simulink model "CFBTTCQIED"  (R2021b)
settings: Solver=ode23t  StartTime=0.0  StopTime=simtime  RelTol=1e-3
values from neighbouring files (symbols this model uses):
  a1 = (Iyy-Izz)/Ixx    (= -0.733333333333)    [CFBTTCQIED.m]
  a1_p = 1    [CFBTTCQIED.m]
  a1_r = 1    [CFBTTCQIED.m]
  a1_x = 1    [CFBTTCQIED.m]
  a1_y = 1    [CFBTTCQIED.m]
  a1_z = 1    [CFBTTCQIED.m]
  a2 = Jr/Ixx    (= 0.008)    [CFBTTCQIED.m]
  a2_r = 2    [CFBTTCQIED.m]
  a2_x = 2    [CFBTTCQIED.m]
  a2_y = 2    [CFBTTCQIED.m]
  a2_z = 2    [CFBTTCQIED.m]
  a3 = (Izz-Ixx)/Iyy    (= 0.733333333333)    [CFBTTCQIED.m]
  a4 = Jr/Iyy    (= 0.008)    [CFBTTCQIED.m]
  a5 = (Ixx-Iyy)/Izz    (= 0)    [CFBTTCQIED.m]
  b = 3.13e-5    (= 3.13e-05)    [CFBTTCQIED.m]
  b1 = l/Ixx    (= 30.6666666667)    [CFBTTCQIED.m]
  b2 = l/Iyy    (= 30.6666666667)    [CFBTTCQIED.m]
  b3 = l/Izz    (= 17.6923076923)    [CFBTTCQIED.m]
  d = 7.5e-7    (= 7.5e-07)    [CFBTTCQIED.m]
  epsi = 0.00001    (= 1e-05)    [CFBTTCQIED.m]
  g = 9.81    [CFBTTCQIED.m]
  init_cond_pitch = 0    [CFBTTCQIED.m]
  init_cond_roll = 0    [CFBTTCQIED.m]
  init_cond_x = 0    [CFBTTCQIED.m]
  init_cond_y = 2    [CFBTTCQIED.m]
  init_cond_yaw = 0    [CFBTTCQIED.m]
  init_cond_z = 0    [CFBTTCQIED.m]
  k = 2.980e-6    (= 2.98e-06)    [CFBTTCQIED.m]
  lambda = zxc    (= 10)    [CFBTTCQIED.m]
  lambda_x = 2    [CFBTTCQIED.m]
  lambda_y = 2    [CFBTTCQIED.m]
  lambda_z = 2    [CFBTTCQIED.m]
  lamda_phi = zxc    (= 10)    [CFBTTCQIED.m]
  lamda_psi = zxc    (= 10)    [CFBTTCQIED.m]
  lamda_theta = zxc    (= 10)    [CFBTTCQIED.m]
  m = 0.650    (= 0.65)    [CFBTTCQIED.m]
  Omega_r = 1    [CFBTTCQIED.m]
  p1_phi = 20    [CFBTTCQIED.m]
  p1_psi = 20    [CFBTTCQIED.m]
  p1_theta = 20    [CFBTTCQIED.m]
  p1_x = 2    [CFBTTCQIED.m]
  p1_y = 2    [CFBTTCQIED.m]
  p1_z = 2    [CFBTTCQIED.m]
  p2_phi = 5    [CFBTTCQIED.m]
  p2_psi = 5    [CFBTTCQIED.m]
  p2_theta = 5    [CFBTTCQIED.m]
  p2_x = 2    [CFBTTCQIED.m]
  p2_y = 2    [CFBTTCQIED.m]
  p2_z = 2    [CFBTTCQIED.m]
  psi_des = yaw_des    (= 0.523598775598)    [CFBTTCQIED.m]
  sample_time_pitch = 15    [CFBTTCQIED.m]
  sample_time_roll = 15    [CFBTTCQIED.m]
  sample_time_yaw = 1    [CFBTTCQIED.m]
  tau = 0.1    [CFBTTCQIED.m]
libraries: simulink x2
(part 1 of 2)
settings Model: Creator=nigarahmed  LastModifiedBy=Nigar

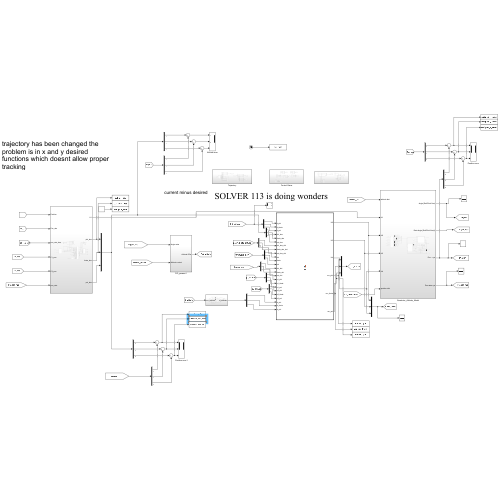
[thumbnail: Simulink's stored preview of the top-level diagram]
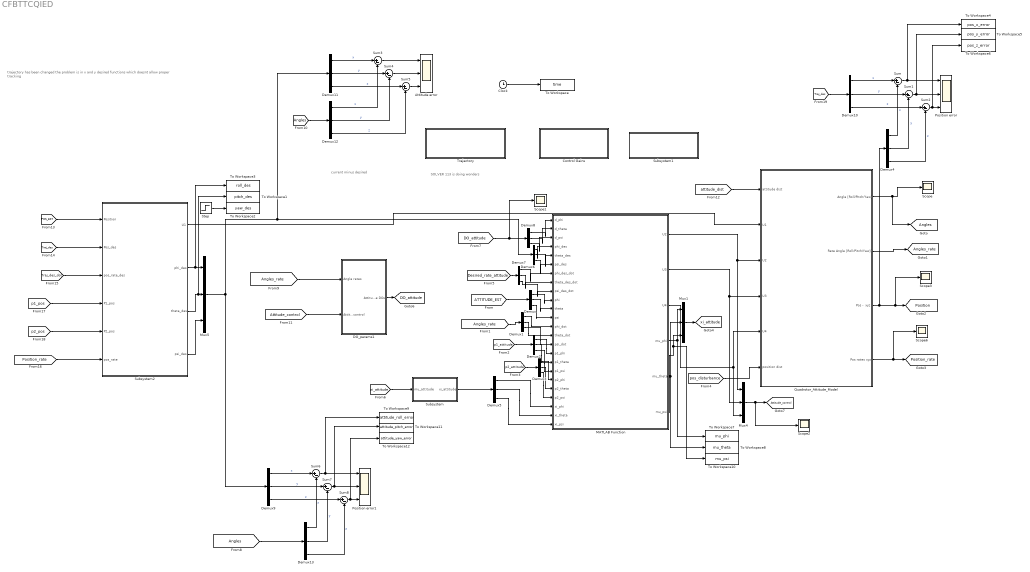
== system CFBTTCQIED ==
  note: current minus desired
  note: SOLVER 113 is doing wonders
  note: trajectory has been changed the problem is in x and y desired functions which doesnt allow proper tracking
  Attitude error : Scope  NumInputPorts=3
  Clock : Clock
  Control Gains : Subsystem
  DO_params1 : Subsystem
  Demux{,1..13} (14 alike) : Demux  Outputs=3
  MATLAB Function : MATLAB Function  TreatAsAtomicUnit=on
  Mux1 : Mux  Inputs=3
  Mux4 : Mux  Inputs=3
  Mux5 : Mux  Inputs=3
  Position error : Scope  NumInputPorts=3
  Position error1 : Scope  NumInputPorts=3
  Quadrotor_Attitude_Model : Subsystem
  Scope{,1..3,6} (5 alike) : Scope
  Step : Step  Time=0  After=psi_des  SampleTime=0
  Subsystem : Subsystem
  Subsystem1 : Subsystem
  Subsystem2 : Subsystem
  Sum{,1..8} (9 alike) : Sum  Inputs=|+-
  To Workspace : ToWorkspace  VariableName=time  SampleTime=-1
  To Workspace1 : ToWorkspace  VariableName=pitch_des  SampleTime=-1
  To Workspace10 : ToWorkspace  VariableName=mu_psi  SampleTime=-1
  To Workspace11 : ToWorkspace  VariableName=attitude_pitch_error  SampleTime=-1
  To Workspace12 : ToWorkspace  VariableName=attitude_yaw_error  SampleTime=-1
  To Workspace2 : ToWorkspace  VariableName=yaw_des  SampleTime=-1
  To Workspace3 : ToWorkspace  VariableName=roll_des  SampleTime=-1
  To Workspace4 : ToWorkspace  VariableName=pos_x_error  SampleTime=-1
  To Workspace5 : ToWorkspace  VariableName=pos_y_error  SampleTime=-1
  To Workspace6 : ToWorkspace  VariableName=pos_z_error  SampleTime=-1
  To Workspace7 : ToWorkspace  VariableName=mu_phi  SampleTime=-1
  To Workspace8 : ToWorkspace  VariableName=mu_theta  SampleTime=-1
  To Workspace9 : ToWorkspace  VariableName=attitude_roll_error  SampleTime=-1
  Trajectory : Subsystem
  tag scope: Angles=global, Angles_rate=global, Attitude_control=global, DO_attitude=global, Position=global, Position_rate=global, xi_attitude=global
  wires:
  [p1_pos] -> Subsystem2/4(P1_pos)
  Quadrotor_Attitude_Model/4(Pos rates xyz) -> Scope6/1, [Position_rate]
  Sum2/1 -> To Workspace6/1, Position error/3
  [Angles_rate] -> DO_params1/1(Angle rates)
  Quadrotor_Attitude_Model/1(Angle [Roll/Pitch/Yaw]) -> [Angles], Scope/1
  DO_params1/1(Attitude DOs) -> [DO_attitude]
  Demux4/3 -> Sum2/2  "z"
  Sum/1 -> To Workspace4/1, Position error/1
  Demux10/2 -> Sum1/1  "y"
  Demux6/2 -> MATLAB Function/5(theta_des)
  [DO_attitude] -> Demux8/1, Scope1/1
  Demux/2 -> MATLAB Function/11(theta)
  Demux4/1 -> Sum/2  "x"
  Demux3/1 -> MATLAB Function/19(p2_phi)
  Demux10/3 -> Sum2/1  "z"
  Demux5/3 -> MATLAB Function/24(xi_psi)
  Demux8/3 -> MATLAB Function/3(d_psi)
  [POS_EST] -> Subsystem2/1(Position)
  Demux6/1 -> MATLAB Function/4(phi_des)
  [Angles_rate] -> Demux1/1
  Demux/1 -> MATLAB Function/10(phi)
  Demux1/3 -> MATLAB Function/15(psi_dot)
  Demux3/2 -> MATLAB Function/20(p2_theta)
  Demux8/1 -> MATLAB Function/1(d_phi)
  Demux6/3 -> MATLAB Function/6(psi_des)
  Demux3/3 -> MATLAB Function/21(p2_psi)
  Subsystem2/4(psi_des) -> Mux5/3
  Subsystem/1(xi_attitude) -> Demux5/1
  Demux5/2 -> MATLAB Function/23(xi_theta)
  Demux2/1 -> MATLAB Function/16(p1_phi)
  Subsystem2/3(theta_des) -> To Workspace1/1, Mux5/2
  Demux8/2 -> MATLAB Function/2(d_theta)
  Mux1/1 -> [xi_attitude]
  Quadrotor_Attitude_Model/2(Rate Angle [Roll/Pitch/Yaw]1) -> [Angles_rate]
  Demux2/2 -> MATLAB Function/17(p1_theta)
  MATLAB Function/5(mu_theta) -> Mux1/2, To Workspace8/1
  MATLAB Function/4(mu_phi) -> Mux1/1, To Workspace7/1
  Quadrotor_Attitude_Model/3(Pos -  xyz) -> Demux4/1, Scope3/1, [Position]
  MATLAB Function/6(mu_psi) -> To Workspace10/1, Mux1/3
  Demux7/2 -> MATLAB Function/8(theta_des_dot)
  Demux/3 -> MATLAB Function/12(psi)
  MATLAB Function/3(U4) -> Mux4/3, Quadrotor_Attitude_Model/5(U4)
  [xi_attitude] -> Subsystem/1(mu_attitude)
  Demux7/1 -> MATLAB Function/7(phi_des_dot)
  [p2_attitude] -> Demux3/1
  Demux1/1 -> MATLAB Function/13(phi_dot)
  [p2_pos] -> Subsystem2/5(P2_pos)
  Demux5/1 -> MATLAB Function/22(xi_phi)
  Demux7/3 -> MATLAB Function/9(psi_des_dot)
  MATLAB Function/1(U2) -> Mux4/1, Quadrotor_Attitude_Model/3(U2)
  Mux4/1 -> Scope2/1, [Attitude_control]
  Subsystem2/1(U1) -> Quadrotor_Attitude_Model/2(U1)
  [attitude_dist] -> Quadrotor_Attitude_Model/1(attitude dist)
  [Traj_des_dot] -> Subsystem2/3(pos_rate_des)
  [Position_rate] -> Subsystem2/6(pos_rate)
  [Traj_des] -> Demux10/1
  MATLAB Function/2(U3) -> Mux4/2, Quadrotor_Attitude_Model/4(U3)
  Demux1/2 -> MATLAB Function/14(theta_dot)
  [p1_attitude] -> Demux2/1
  [Attitude_control] -> DO_params1/2(Attitude control)
  Subsystem2/2(phi_des) -> To Workspace3/1, Mux5/1
  [ATTITUDE_EST] -> Demux/1
  Demux10/1 -> Sum/1  "x"
  Demux4/2 -> Sum1/2  "y"
  [Traj_des] -> Subsystem2/2(Pos_des)
  Sum1/1 -> To Workspace5/1, Position error/2
  [Desired_rate_attitude] -> Demux7/1
  Demux2/3 -> MATLAB Function/18(p1_psi)
  Clock/1 -> To Workspace/1
  Step/1 -> To Workspace2/1
  Demux11/3 -> Sum5/1  "z"
  Sum3/1 -> Attitude error/1
  Demux11/2 -> Sum4/1  "y"
  Sum5/1 -> Attitude error/3
  Demux11/1 -> Sum3/1  "x"
  Sum4/1 -> Attitude error/2
  Demux12/1 -> Sum3/2  "x"
  Demux12/2 -> Sum4/2  "y"
  Demux12/3 -> Sum5/2  "z"
  [Angles] -> Demux12/1
  [pos_disturbance] -> Quadrotor_Attitude_Model/6(position dist)
  Demux9/3 -> Sum8/1  "z"
  Sum6/1 -> To Workspace9/1, Position error1/1
  Sum8/1 -> To Workspace12/1, Position error1/3
  Demux13/3 -> Sum8/2  "z"
  Sum7/1 -> To Workspace11/1, Position error1/2
  Demux13/2 -> Sum7/2  "y"
  Mux5/1 -> Demux6/1, Demux11/1, Demux9/1
  Demux9/2 -> Sum7/1  "y"
  Demux13/1 -> Sum6/2  "x"
  Demux9/1 -> Sum6/1  "x"
  [Angles] -> Demux13/1

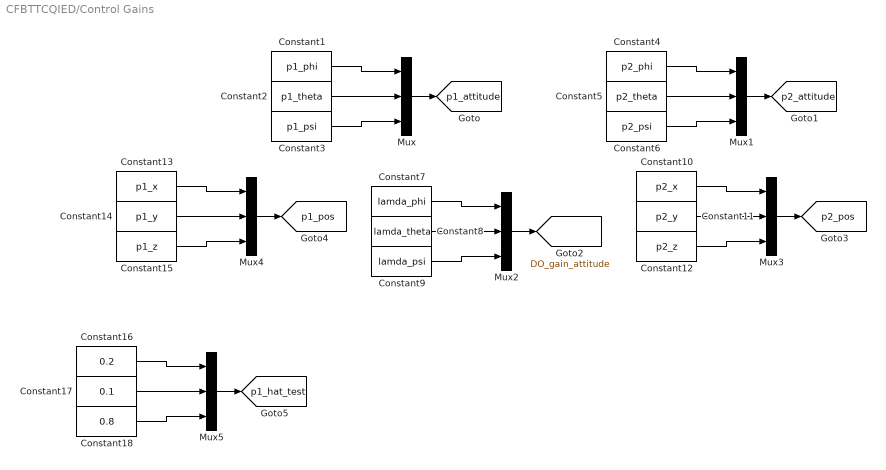
== system CFBTTCQIED/Control Gains ==
  Constant1 : Constant  Value=p1_phi
  Constant10 : Constant  Value=p2_x
  Constant11 : Constant  Value=p2_y
  Constant12 : Constant  Value=p2_z
  Constant13 : Constant  Value=p1_x
  Constant14 : Constant  Value=p1_y
  Constant15 : Constant  Value=p1_z
  Constant16 : Constant  Value=0.2
  Constant17 : Constant  Value=0.1
  Constant18 : Constant  Value=0.8
  Constant2 : Constant  Value=p1_theta
  Constant3 : Constant  Value=p1_psi
  Constant4 : Constant  Value=p2_phi
  Constant5 : Constant  Value=p2_theta
  Constant6 : Constant  Value=p2_psi
  Constant7 : Constant  Value=lamda_phi
  Constant8 : Constant  Value=lamda_theta
  Constant9 : Constant  Value=lamda_psi
  Mux{,1..5} (6 alike) : Mux  Inputs=3
  tag scope: DO_gain_attitude=global, p1_attitude=global, p1_hat_test=global, p1_pos=global, p2_attitude=global, p2_pos=global
  wires:
  Constant1/1 -> Mux/1
  Constant2/1 -> Mux/2
  Constant3/1 -> Mux/3
  Mux/1 -> [p1_attitude]
  Constant6/1 -> Mux1/3
  Mux1/1 -> [p2_attitude]
  Constant5/1 -> Mux1/2
  Constant4/1 -> Mux1/1
  Constant9/1 -> Mux2/3
  Constant8/1 -> Mux2/2
  Mux2/1 -> [DO_gain_attitude]
  Constant7/1 -> Mux2/1
  Mux3/1 -> [p2_pos]
  Constant12/1 -> Mux3/3
  Constant11/1 -> Mux3/2
  Constant10/1 -> Mux3/1
  Mux4/1 -> [p1_pos]
  Constant15/1 -> Mux4/3
  Constant14/1 -> Mux4/2
  Constant13/1 -> Mux4/1
  Constant18/1 -> Mux5/3
  Constant17/1 -> Mux5/2
  Constant16/1 -> Mux5/1
  Mux5/1 -> [p1_hat_test]

== system CFBTTCQIED/DO_params1 ==
  Angle rates : Inport
  Attitude control : Inport  Port=2
  Demux : Demux  Outputs=3
  Demux1 : Demux  Outputs=3
  Mux1 : Mux  Inputs=3
  Pitch DO : Subsystem
  Pitch DO1 : Subsystem
  "ROLL DO " : Subsystem
  To Workspace : ToWorkspace  VariableName=roll_DO  SaveFormat=Timeseries  SampleTime=-1
  To Workspace1 : ToWorkspace  VariableName=pitch_DO  SaveFormat=Timeseries  SampleTime=-1
  To Workspace2 : ToWorkspace  VariableName=yaw_DO  SaveFormat=Timeseries  SampleTime=-1
  Attitude DOs : Outport
  wires:
  Mux1/1 -> Attitude DOs/1
  "ROLL DO "/1(ROLL DO) -> To Workspace/1, Mux1/1
  Pitch DO/1(Pitch DO) -> To Workspace1/1, Mux1/2
  Pitch DO1/1(Yaw DOs) -> Mux1/3, To Workspace2/1
  Demux/1 -> Pitch DO1/1(phi_dot), Pitch DO/1(phi_dot), "ROLL DO "/1(phi_dot)
  Demux/2 -> Pitch DO1/2(theta_dot), Pitch DO/2(theta_dot), "ROLL DO "/2(theta_dot)
  Demux/3 -> Pitch DO1/3(psi_dot), Pitch DO/3(psi_dot), "ROLL DO "/3(psi_dot)
  Demux1/1 -> "ROLL DO "/4(U2)
  Demux1/2 -> Pitch DO/4(U3)
  Demux1/3 -> Pitch DO1/4(U4)
  Angle rates/1 -> Demux/1
  Attitude control/1 -> Demux1/1

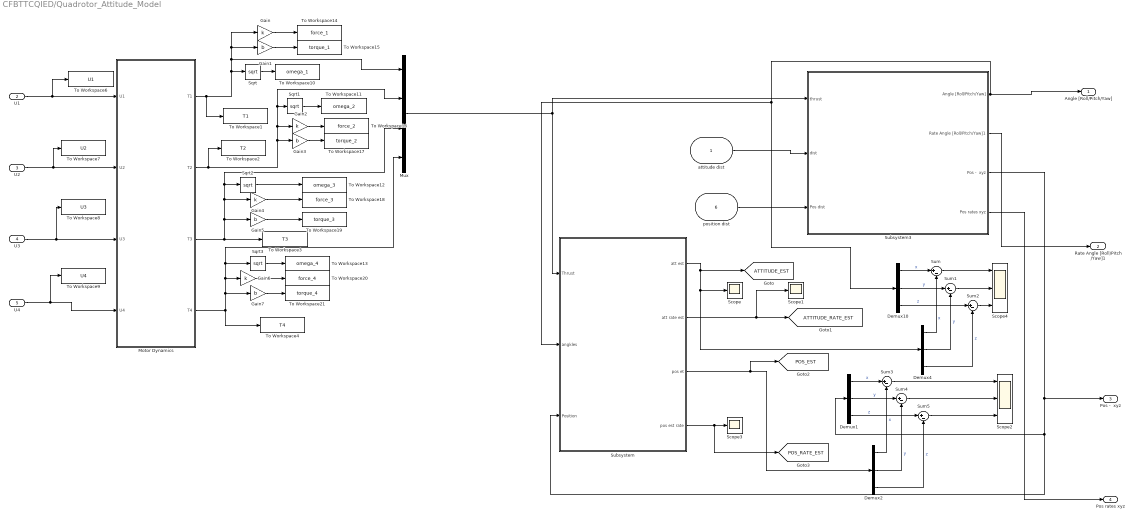
== system CFBTTCQIED/Quadrotor_Attitude_Model ==
  attitude dist : Inport
  U1 : Inport  Port=2
  U2 : Inport  Port=3
  U3 : Inport  Port=4
  U4 : Inport  Port=5
  position dist : Inport  Port=6
  Demux{1..2,4,10} (4 alike) : Demux  Outputs=3
  Gain{,2,4,6} (4 alike) : Gain  Gain=k
  Gain{1,3,5,7} (4 alike) : Gain  Gain=b
  Motor Dynamics : MATLAB Function  TreatAsAtomicUnit=on
  Mux : Mux
  Scope : Scope
  Scope1 : Scope
  Scope2 : Scope  NumInputPorts=3
  Scope3 : Scope
  Scope4 : Scope  NumInputPorts=3
  Sqrt{,1..3} (4 alike) : Sqrt  SaturateOnIntegerOverflow=on
  Subsystem : Subsystem
  Subsystem3 : Subsystem
  Sum{,1..5} (6 alike) : Sum  Inputs=|+-
  To Workspace1 : ToWorkspace  VariableName=T1  SampleTime=-1
  To Workspace10 : ToWorkspace  VariableName=omega_1  SampleTime=-1
  To Workspace11 : ToWorkspace  VariableName=omega_2  SampleTime=-1
  To Workspace12 : ToWorkspace  VariableName=omega_3  SampleTime=-1
  To Workspace13 : ToWorkspace  VariableName=omega_4  SampleTime=-1
  To Workspace14 : ToWorkspace  VariableName=force_1  SampleTime=-1
  To Workspace15 : ToWorkspace  VariableName=torque_1  SampleTime=-1
  To Workspace16 : ToWorkspace  VariableName=force_2  SampleTime=-1
  To Workspace17 : ToWorkspace  VariableName=torque_2  SampleTime=-1
  To Workspace18 : ToWorkspace  VariableName=force_3  SampleTime=-1
  To Workspace19 : ToWorkspace  VariableName=torque_3  SampleTime=-1
  To Workspace2 : ToWorkspace  VariableName=T2  SampleTime=-1
  To Workspace20 : ToWorkspace  VariableName=force_4  SampleTime=-1
  To Workspace21 : ToWorkspace  VariableName=torque_4  SampleTime=-1
  To Workspace3 : ToWorkspace  VariableName=T3  SampleTime=-1
  To Workspace4 : ToWorkspace  VariableName=T4  SampleTime=-1
  To Workspace6 : ToWorkspace  VariableName=U1  SampleTime=-1
  To Workspace7 : ToWorkspace  VariableName=U2  SampleTime=-1
  To Workspace8 : ToWorkspace  VariableName=U3  SampleTime=-1
  To Workspace9 : ToWorkspace  VariableName=U4  SampleTime=-1
  Angle [Roll/Pitch/Yaw] : Outport
  Rate Angle [Roll/Pitch/Yaw]1 : Outport  Port=2
  Pos -  xyz : Outport  Port=3
  Pos rates xyz : Outport  Port=4
  tag scope: ATTITUDE_EST=global, ATTITUDE_RATE_EST=global, POS_EST=global, POS_RATE_EST=global
  wires:
  Motor Dynamics/2(T2) -> To Workspace2/1, Mux/2, Sqrt1/1, Gain2/1, Gain3/1
  Motor Dynamics/4(T4) -> Mux/4, Sqrt3/1, Gain6/1, Gain7/1, To Workspace4/1
  Motor Dynamics/1(T1) -> Gain1/1, Gain/1, Mux/1, Sqrt/1, To Workspace1/1
  Motor Dynamics/3(T3) -> To Workspace3/1, Mux/3, Sqrt2/1, Gain4/1, Gain5/1
  U1/1 -> To Workspace6/1, Motor Dynamics/1(U1)
  U2/1 -> To Workspace7/1, Motor Dynamics/2(U2)
  U3/1 -> To Workspace8/1, Motor Dynamics/3(U3)
  U4/1 -> To Workspace9/1, Motor Dynamics/4(U4)
  Sqrt/1 -> To Workspace10/1
  Sqrt1/1 -> To Workspace11/1
  Sqrt2/1 -> To Workspace12/1
  Sqrt3/1 -> To Workspace13/1
  Gain/1 -> To Workspace14/1
  Gain1/1 -> To Workspace15/1
  Gain2/1 -> To Workspace16/1
  Gain3/1 -> To Workspace17/1
  Gain4/1 -> To Workspace18/1
  Gain5/1 -> To Workspace19/1
  Gain6/1 -> To Workspace20/1
  Gain7/1 -> To Workspace21/1
  Subsystem3/1(Angle [Roll/Pitch/Yaw]) -> Subsystem/2(angkles), Demux10/1, Angle [Roll/Pitch/Yaw]/1
  Subsystem3/2(Rate Angle [Roll/Pitch/Yaw]1) -> Rate Angle [Roll/Pitch/Yaw]1/1
  Subsystem3/3(Pos -  xyz) -> Subsystem/3(Position), Demux1/1, Pos -  xyz/1
  Subsystem3/4(Pos rates xyz) -> Pos rates xyz/1
  attitude dist/1 -> Subsystem3/2(dist)
  Mux/1 -> Subsystem/1(Thrust), Subsystem3/1(thrust)
  Subsystem/1(att est) -> Demux4/1, Scope/1, [ATTITUDE_EST]
  Subsystem/2(att rate est) -> Scope1/1, [ATTITUDE_RATE_EST]
  Sum/1 -> Scope4/1
  Sum1/1 -> Scope4/2
  Demux4/3 -> Sum2/2  "z"
  Demux4/1 -> Sum/2  "x"
  Sum2/1 -> Scope4/3
  Demux10/1 -> Sum/1  "x"
  Demux10/3 -> Sum2/1  "z"
  Demux4/2 -> Sum1/2  "y"
  Demux10/2 -> Sum1/1  "y"
  Demux2/2 -> Sum4/2  "y"
  Demux1/1 -> Sum3/1  "x"
  Demux1/3 -> Sum5/1  "z"
  Demux1/2 -> Sum4/1  "y"
  Sum5/1 -> Scope2/3
  Demux2/3 -> Sum5/2  "z"
  Sum4/1 -> Scope2/2
  Sum3/1 -> Scope2/1
  Demux2/1 -> Sum3/2  "x"
  Subsystem/3(pos et) -> [POS_EST], Demux2/1
  Subsystem/4(pos est rate) -> [POS_RATE_EST], Scope3/1
  position dist/1 -> Subsystem3/3(Pos dist)

== system CFBTTCQIED/Subsystem ==
  mu_attitude : Inport
  Demux : Demux  Outputs=3
  Gain{,1..5} (6 alike) : Gain  Gain=1/tau
  Integrator : Integrator
  Integrator1 : Integrator
  Integrator2 : Integrator
  Mux : Mux  Inputs=3
  Sum{,1..5} (6 alike) : Sum  Inputs=|+-
  To Workspace : ToWorkspace  VariableName=filter_1  SampleTime=-1
  To Workspace1 : ToWorkspace  VariableName=filter_2  SampleTime=-1
  To Workspace2 : ToWorkspace  VariableName=filter_3  SampleTime=-1
  xi_attitude : Outport
  wires:
  Integrator/1 -> To Workspace/1, Sum3/2, Sum/2
  Sum/1 -> Gain/1
  Gain/1 -> Integrator/1
  Sum1/1 -> Gain1/1
  Gain1/1 -> Integrator1/1
  Demux/2 -> Sum4/1, Sum1/1
  Integrator1/1 -> Sum4/2, Sum1/2, To Workspace1/1
  Sum2/1 -> Gain2/1
  Gain2/1 -> Integrator2/1
  Demux/3 -> Sum5/1, Sum2/1
  Demux/1 -> Sum3/1, Sum/1
  mu_attitude/1 -> Demux/1
  Mux/1 -> xi_attitude/1
  Sum3/1 -> Gain3/1
  Gain3/1 -> Mux/1
  Sum4/1 -> Gain4/1
  Gain4/1 -> Mux/2
  Gain5/1 -> Mux/3
  Sum5/1 -> Gain5/1
  Integrator2/1 -> Sum2/2, To Workspace2/1, Sum5/2

== system CFBTTCQIED/Subsystem1 ==
  Band-Limited White Noise : simulink/Sources/Band-Limited White Noise  Cov=[0.05]  Ts=sample_time_yaw  seed=[23341]
  Chirp Signal : simulink/Sources/Chirp Signal  f1=0.01  T=100  f2=0.001
  Mux1 : Mux  Inputs=3
  Mux5 : Mux  Inputs=3
  Random Number : RandomNumber  Mean=0.75  Variance=0.1  Seed=1  SampleTime=sample_time_roll
  Scope : Scope
  Sine Wave : Sin  Frequency=0.1  SampleTime=0
  Step2 : Step  Time=50  ZeroCross=off
  To Workspace : ToWorkspace  VariableName=roll_dist  SaveFormat=Timeseries  SampleTime=-1
  To Workspace1 : ToWorkspace  VariableName=pitch_dist  SaveFormat=Timeseries  SampleTime=-1
  To Workspace2 : ToWorkspace  VariableName=yaw_dist  SaveFormat=Timeseries  SampleTime=-1
  To Workspace3 : ToWorkspace  VariableName=pos_x_dist  SampleTime=-1
  To Workspace4 : ToWorkspace  VariableName=pos_y_dist  SaveFormat=Timeseries  SampleTime=-1
  To Workspace5 : ToWorkspace  VariableName=pos_z_dist  SaveFormat=Timeseries  SampleTime=-1
  Uniform Random Number : UniformRandomNumber  Minimum=-0.5  Maximum=0.5  Seed=0.5  SampleTime=sample_time_pitch
  tag scope: attitude_dist=global, pos_disturbance=global
  wires:
  Uniform Random Number/1 -> To Workspace1/1, Mux1/2
  Step2/1 -> To Workspace4/1, Mux5/2
  Mux1/1 -> [attitude_dist]
  Random Number/1 -> To Workspace/1, Mux1/1
  Mux5/1 -> [pos_disturbance]
  Band-Limited White Noise/1 -> To Workspace2/1, Scope/1, Mux1/3
  Chirp Signal/1 -> Mux5/3, To Workspace5/1
  Sine Wave/1 -> To Workspace3/1, Mux5/1

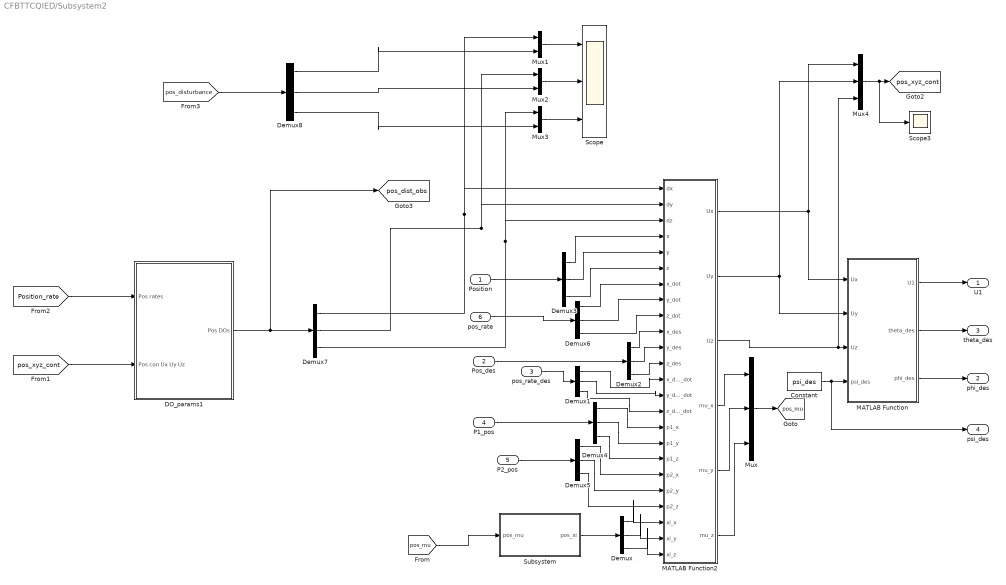
== system CFBTTCQIED/Subsystem2 ==
  Position : Inport
  Pos_des : Inport  Port=2
  pos_rate_des : Inport  Port=3
  P1_pos : Inport  Port=4
  P2_pos : Inport  Port=5
  pos_rate : Inport  Port=6
  Constant : Constant  Value=psi_des
  DO_params1 : Subsystem
  Demux{,1..8} (9 alike) : Demux  Outputs=3
  MATLAB Function : MATLAB Function  TreatAsAtomicUnit=on
  MATLAB Function2 : MATLAB Function  TreatAsAtomicUnit=on
  Mux : Mux  Inputs=3
  Mux1 : Mux  Inputs=2
  Mux2 : Mux  Inputs=2
  Mux3 : Mux  Inputs=2
  Mux4 : Mux  Inputs=3
  Scope : Scope  NumInputPorts=3
  Scope3 : Scope
  Subsystem : Subsystem
  U1 : Outport
  phi_des : Outport  Port=2
  theta_des : Outport  Port=3
  psi_des : Outport  Port=4
  tag scope: pos_dist_obs=global, pos_mu=global, pos_xyz_cont=global
  wires:
  MATLAB Function2/1(Ux) -> Mux4/1, MATLAB Function/1(Ux)
  MATLAB Function2/2(Uy) -> Mux4/2, MATLAB Function/2(Uy)
  MATLAB Function2/3(Uz) -> Mux4/3, MATLAB Function/3(Uz)
  Constant/1 -> psi_des/1, MATLAB Function/4(psi_des)
  MATLAB Function2/4(mu_x) -> Mux/1
  MATLAB Function2/5(mu_y) -> Mux/2
  MATLAB Function2/6(mu_z) -> Mux/3
  Mux/1 -> [pos_mu]
  Demux/1 -> MATLAB Function2/22(xi_x)
  Demux/2 -> MATLAB Function2/23(xi_y)
  Demux/3 -> MATLAB Function2/24(xi_z)
  Subsystem/1(pos_xi) -> Demux/1
  [pos_mu] -> Subsystem/1(pos_mu)
  Demux1/2 -> MATLAB Function2/14(y_des_dot)
  Demux1/3 -> MATLAB Function2/15(z_des_dot)
  Demux1/1 -> MATLAB Function2/13(x_des_dot)
  pos_rate_des/1 -> Demux1/1
  Demux2/1 -> MATLAB Function2/10(x_des)
  Demux2/2 -> MATLAB Function2/11(y_des)
  Demux2/3 -> MATLAB Function2/12(z_des)
  Pos_des/1 -> Demux2/1
  Demux3/1 -> MATLAB Function2/4(x)
  Demux3/2 -> MATLAB Function2/5(y)
  Demux3/3 -> MATLAB Function2/6(z)
  Position/1 -> Demux3/1
  MATLAB Function/1(U1) -> U1/1
  MATLAB Function/2(theta_des) -> theta_des/1
  MATLAB Function/3(phi_des) -> phi_des/1
  Demux4/1 -> MATLAB Function2/16(p1_x)
  Demux4/2 -> MATLAB Function2/17(p1_y)
  Demux4/3 -> MATLAB Function2/18(p1_z)
  Demux5/3 -> MATLAB Function2/21(p2_z)
  Demux5/2 -> MATLAB Function2/20(p2_y)
  Demux5/1 -> MATLAB Function2/19(p2_x)
  P1_pos/1 -> Demux4/1
  P2_pos/1 -> Demux5/1
  pos_rate/1 -> Demux6/1
  Demux6/1 -> MATLAB Function2/7(x_dot)
  Demux6/2 -> MATLAB Function2/8(y_dot)
  Demux6/3 -> MATLAB Function2/9(z_dot)
  [Position_rate] -> DO_params1/1(Pos rates)
  DO_params1/1(Pos DOs) -> Demux7/1, [pos_dist_obs]
  [pos_xyz_cont] -> DO_params1/2(Pos con Ux Uy Uz)
  Demux7/1 -> MATLAB Function2/1(dx), Mux1/1
  Demux7/2 -> MATLAB Function2/2(dy), Mux2/1
  Demux7/3 -> MATLAB Function2/3(dz), Mux3/1
  Mux1/1 -> Scope/1
  Mux2/1 -> Scope/2
  Mux3/1 -> Scope/3
  [pos_disturbance] -> Demux8/1
  Demux8/1 -> Mux1/2
  Demux8/2 -> Mux2/2
  Demux8/3 -> Mux3/2
  Mux4/1 -> Scope3/1, [pos_xyz_cont]

== system CFBTTCQIED/Trajectory ==
  Clock : Clock
  Demux : Demux  Outputs=3
  Derivative{,1..5} (6 alike) : Derivative
  MATLAB Function2 : MATLAB Function  TreatAsAtomicUnit=on
  Mux{,1..3} (4 alike) : Mux  Inputs=3
  To Workspace : ToWorkspace  VariableName=x_des  SampleTime=-1
  To Workspace1 : ToWorkspace  VariableName=y_des  SampleTime=-1
  To Workspace2 : ToWorkspace  VariableName=z_des  SampleTime=-1
  tag scope: Desired_attitude=global, Desired_rate_attitude=global, Traj_des=global, Traj_des_dot=global
  wires:
  MATLAB Function2/1(x_des) -> To Workspace/1, Mux/1, Derivative/1
  Clock/1 -> MATLAB Function2/1(t)
  MATLAB Function2/2(y_des) -> To Workspace1/1, Mux/2, Derivative1/1
  MATLAB Function2/3(z_des) -> Derivative2/1, Mux/3, To Workspace2/1
  Mux/1 -> [Traj_des]
  Derivative/1 -> Mux1/1
  Derivative1/1 -> Mux1/2
  Derivative2/1 -> Mux1/3
  Mux1/1 -> [Traj_des_dot]
  Demux/1 -> Derivative3/1, Mux2/1
  Demux/2 -> Mux2/2, Derivative4/1
  Demux/3 -> Mux2/3, Derivative5/1
  Mux2/1 -> [Desired_attitude]
  Mux3/1 -> [Desired_rate_attitude]
  Derivative3/1 -> Mux3/1
  Derivative4/1 -> Mux3/2
  Derivative5/1 -> Mux3/3
  [Desired_attitude_pos] -> Demux/1

== system CFBTTCQIED/DO_params1/Pitch DO ==
  phi_dot : Inport
  theta_dot : Inport  Port=2
  psi_dot : Inport  Port=3
  U3 : Inport  Port=4
  Gain1 : Gain  Gain=a3
  Gain2 : Gain  Gain=a4*Omega_r
  Gain{4,6..7,9} (4 alike) : Gain  Gain=lambda
  Gain5 : Gain  Gain=lambda*lambda
  Gain8 : Gain  Gain=lambda*b2
  Integrator2 : Integrator
  Product : Product
  Sum1 : Sum
  Sum4 : Sum  Inputs=---+-
  Pitch DO : Outport
  wires:
  Sum1/1 -> Pitch DO/1
  Gain9/1 -> Sum1/2
  Integrator2/1 -> Gain4/1, Sum1/1
  Sum4/1 -> Integrator2/1
  Gain8/1 -> Sum4/5
  Gain7/1 -> Sum4/4
  Gain6/1 -> Sum4/3
  Gain5/1 -> Sum4/2
  Gain4/1 -> Sum4/1
  Product/1 -> Gain1/1
  Gain1/1 -> Gain6/1
  Gain2/1 -> Gain7/1
  theta_dot/1 -> Gain9/1, Gain5/1
  phi_dot/1 -> Gain2/1, Product/1
  psi_dot/1 -> Product/2
  U3/1 -> Gain8/1

== system CFBTTCQIED/DO_params1/Pitch DO1 ==
  phi_dot : Inport
  theta_dot : Inport  Port=2
  psi_dot : Inport  Port=3
  U4 : Inport  Port=4
  Gain1 : Gain  Gain=a5
  Gain4 : Gain  Gain=lambda
  Gain5 : Gain  Gain=lambda*lambda
  Gain6 : Gain  Gain=lambda
  Gain8 : Gain  Gain=lambda*b3
  Gain9 : Gain  Gain=lambda
  Integrator2 : Integrator
  Product : Product
  Sum1 : Sum
  Sum4 : Sum  Inputs=----
  Yaw DOs : Outport
  wires:
  Gain1/1 -> Gain6/1
  Product/1 -> Gain1/1
  Gain4/1 -> Sum4/1
  Gain5/1 -> Sum4/2
  Gain6/1 -> Sum4/3
  Gain8/1 -> Sum4/4
  Sum4/1 -> Integrator2/1
  Integrator2/1 -> Sum1/1, Gain4/1
  Gain9/1 -> Sum1/2
  Sum1/1 -> Yaw DOs/1
  U4/1 -> Gain8/1
  psi_dot/1 -> Gain9/1, Gain5/1
  phi_dot/1 -> Product/1
  theta_dot/1 -> Product/2

== system CFBTTCQIED/DO_params1/ROLL DO  ==
  phi_dot : Inport
  theta_dot : Inport  Port=2
  psi_dot : Inport  Port=3
  U2 : Inport  Port=4
  Gain1 : Gain  Gain=a1
  Gain2 : Gain  Gain=a2*Omega_r
  Gain{4,6..7,9} (4 alike) : Gain  Gain=lambda
  Gain5 : Gain  Gain=lambda*lambda
  Gain8 : Gain  Gain=lambda*b1
  Integrator2 : Integrator
  Product : Product
  Sum1 : Sum
  Sum4 : Sum  Inputs=-----
  ROLL DO : Outport
  wires:
  Gain2/1 -> Gain7/1
  Gain1/1 -> Gain6/1
  phi_dot/1 -> Gain9/1, Gain5/1
  Product/1 -> Gain1/1
  theta_dot/1 -> Gain2/1, Product/1
  Gain4/1 -> Sum4/1
  Gain5/1 -> Sum4/2
  Gain6/1 -> Sum4/3
  Gain7/1 -> Sum4/4
  Gain8/1 -> Sum4/5
  Sum4/1 -> Integrator2/1
  Integrator2/1 -> Sum1/1, Gain4/1
  Gain9/1 -> Sum1/2
  Sum1/1 -> ROLL DO/1
  psi_dot/1 -> Product/2
  U2/1 -> Gain8/1

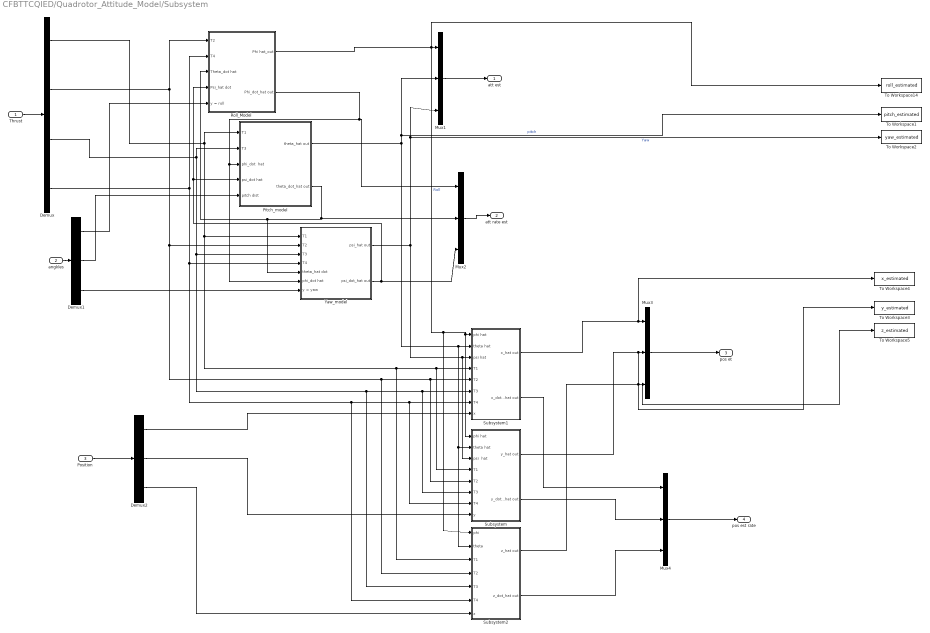
== system CFBTTCQIED/Quadrotor_Attitude_Model/Subsystem ==
  Thrust : Inport
  angkles : Inport  Port=2
  Position : Inport  Port=3
  Demux : Demux
  Demux1 : Demux  Outputs=3
  Demux2 : Demux  Outputs=3
  Mux{1..4} (4 alike) : Mux  Inputs=3
  Pitch_model : Subsystem
  Roll_Model : Subsystem
  Subsystem : Subsystem
  Subsystem1 : Subsystem
  Subsystem2 : Subsystem
  To Workspace1 : ToWorkspace  VariableName=pitch_estimated  SampleTime=-1
  To Workspace14 : ToWorkspace  VariableName=roll_estimated  SampleTime=-1
  To Workspace2 : ToWorkspace  VariableName=yaw_estimated  SampleTime=-1
  To Workspace3 : ToWorkspace  VariableName=y_estimated  SampleTime=-1
  To Workspace4 : ToWorkspace  VariableName=x_estimated  SampleTime=-1
  To Workspace5 : ToWorkspace  VariableName=z_estimated  SampleTime=-1
  Yaw_model : Subsystem
  att est : Outport
  att rate est : Outport  Port=2
  pos et : Outport  Port=3
  pos est rate : Outport  Port=4
  wires:
  Demux/4 -> Yaw_model/4(T4), Subsystem1/7(T4), Subsystem/7(T4), Subsystem2/6(T4), Roll_Model/2(T4)
  angkles/1 -> Demux1/1
  Demux1/1 -> Roll_Model/5(y = roll)
  Demux/1 -> Yaw_model/1(" T1"), Subsystem1/4(T1), Subsystem/4(T1), Subsystem2/3(T1), Pitch_model/1(T1)
  Mux1/1 -> att est/1
  Demux/3 -> Yaw_model/3(T3), Subsystem1/6(T3), Subsystem/6(T3), Subsystem2/5(T3), Pitch_model/2(T3)
  Pitch_model/2(theta_dot_hat out) -> Yaw_model/5("theta_hat dot "), Roll_Model/3("Theta_dot hat "), Mux2/2
  Yaw_model/2(psi_dot_hat out) -> Pitch_model/4("psi_dot hat "), Roll_Model/4("Psi_hat dot "), Mux2/3
  Roll_Model/2(Phi_dot_hat out) -> Yaw_model/6("phi_dot hat  "), Pitch_model/3(phi_dot  hat), Mux2/1
  Demux/2 -> Yaw_model/2(T2), Subsystem2/4(T2), Subsystem1/5(T2), Subsystem/5(T2), Roll_Model/1(T2)
  Roll_Model/1(Phi hat_out) -> Subsystem/1(phi hat), Subsystem1/1(phi hat), Subsystem2/1(phi), Mux1/1, To Workspace14/1  "Roll"
  Demux1/2 -> Pitch_model/5(pitch dist)
  Demux1/3 -> Yaw_model/7(y = yaw)
  Thrust/1 -> Demux/1
  Yaw_model/1(psi_hat out) -> Mux1/3, To Workspace2/1, Subsystem1/3(psi hat), Subsystem/3(psi  hat)  "Yaw"
  Pitch_model/1(theta_hat out) -> Mux1/2, To Workspace1/1, Subsystem/2(theta hat), Subsystem2/2(theta), Subsystem1/2(theta hat)  "pitch"
  Mux2/1 -> att rate est/1
  Mux3/1 -> pos et/1
  Mux4/1 -> pos est rate/1
  Subsystem1/1(x_hat out) -> To Workspace4/1, Mux3/1
  Subsystem/1(y_hat out) -> To Workspace3/1, Mux3/2
  Subsystem2/1(z_hat out) -> To Workspace5/1, Mux3/3
  Subsystem1/2(x_dot_hat out) -> Mux4/1
  Subsystem/2(y_dot_hat out) -> Mux4/2
  Subsystem2/2(z_dot_hat out) -> Mux4/3
  Position/1 -> Demux2/1
  Demux2/1 -> Subsystem1/8(x)
  Demux2/2 -> Subsystem/8(y)
  Demux2/3 -> Subsystem2/7(z)

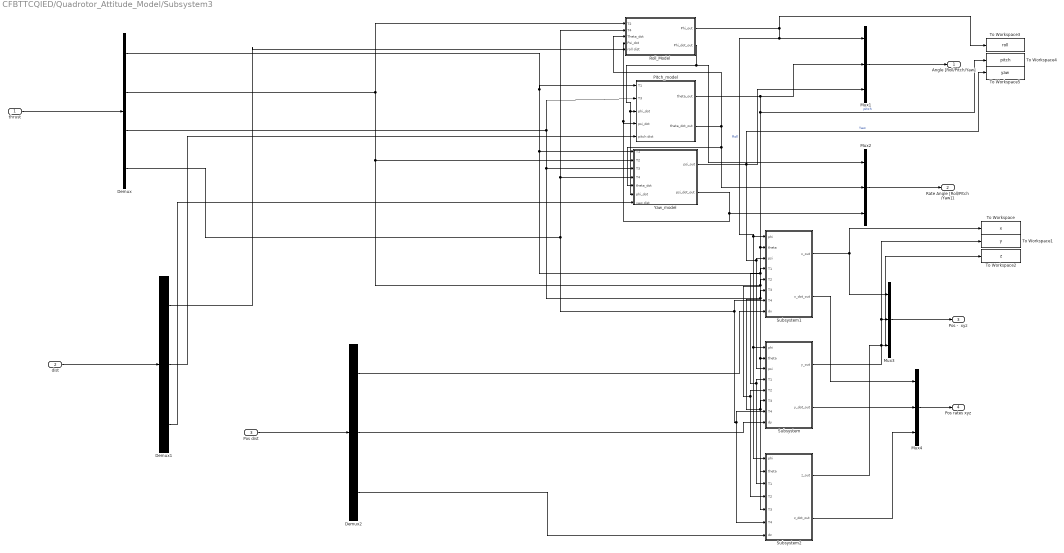
== system CFBTTCQIED/Quadrotor_Attitude_Model/Subsystem3 ==
  thrust : Inport
  dist : Inport  Port=2
  Pos dist : Inport  Port=3
  Demux : Demux
  Demux1 : Demux  Outputs=3
  Demux2 : Demux  Outputs=3
  Mux{1..4} (4 alike) : Mux  Inputs=3
  Pitch_model : Subsystem
  Roll_Model : Subsystem
  Subsystem : Subsystem
  Subsystem1 : Subsystem
  Subsystem2 : Subsystem
  To Workspace : ToWorkspace  VariableName=x  SampleTime=-1
  To Workspace1 : ToWorkspace  VariableName=y  SampleTime=-1
  To Workspace2 : ToWorkspace  VariableName=z  SampleTime=-1
  To Workspace3 : ToWorkspace  VariableName=roll  SampleTime=-1
  To Workspace4 : ToWorkspace  VariableName=pitch  SampleTime=-1
  To Workspace5 : ToWorkspace  VariableName=yaw  SampleTime=-1
  Yaw_model : Subsystem
  Angle [Roll/Pitch/Yaw] : Outport
  Rate Angle [Roll/Pitch/Yaw]1 : Outport  Port=2
  Pos -  xyz : Outport  Port=3
  Pos rates xyz : Outport  Port=4
  wires:
  Demux/3 -> Subsystem2/5(T3), Subsystem/6(T3), Subsystem1/6(T3), Yaw_model/3(T3), Pitch_model/2(T3)
  Yaw_model/2(psi_dot_out) -> Mux2/3, Roll_Model/4("Psi_dot "), Pitch_model/4("psi_dot ")
  Demux/1 -> Subsystem/4(T1), Subsystem2/3(T1), Subsystem1/4(T1), Yaw_model/1(" T1"), Pitch_model/1(T1)
  Subsystem1/1(x_out) -> To Workspace/1, Mux3/1
  Subsystem/2(y_dot_out) -> Mux4/2
  Pitch_model/1(theta_out) -> Subsystem2/2(theta), Subsystem/2(theta), Subsystem1/2(theta), To Workspace4/1, Mux1/2  "pitch"
  Mux3/1 -> Pos -  xyz/1
  Subsystem2/2(z_dot_out) -> Mux4/3
  Roll_Model/1(Phi_out) -> Subsystem1/1(phi), Subsystem/1(phi), Subsystem2/1(phi), Mux1/1, To Workspace3/1  "Roll"
  Subsystem2/1(z_out) -> To Workspace2/1, Mux3/3
  Subsystem1/2(x_dot_out) -> Mux4/1
  Demux/2 -> Subsystem/5(T2), Subsystem2/4(T2), Subsystem1/5(T2), Yaw_model/2(T2), Roll_Model/1(T2)
  Roll_Model/2(Phi_dot_out) -> Mux2/1, Yaw_model/6("phi_dot "), Pitch_model/3("phi_dot ")
  Yaw_model/1(psi_out) -> Mux1/3, Subsystem1/3(psi), Subsystem/3(psi), To Workspace5/1  "Yaw"
  Mux1/1 -> Angle [Roll/Pitch/Yaw]/1
  Mux4/1 -> Pos rates xyz/1
  Mux2/1 -> Rate Angle [Roll/Pitch/Yaw]1/1
  Subsystem/1(y_out) -> To Workspace1/1, Mux3/2
  Pitch_model/2(theta_dot_out) -> Yaw_model/5("theta_dot "), Mux2/2, Roll_Model/3("Theta_dot ")
  Demux/4 -> Subsystem1/7(T4), Subsystem/7(T4), Subsystem2/6(T4), Roll_Model/2(T4), Yaw_model/4(T4)
  Demux1/1 -> Roll_Model/5(roll dist)
  Demux1/3 -> Yaw_model/7(yaw dist)
  Demux1/2 -> Pitch_model/5(pitch dist)
  thrust/1 -> Demux/1
  dist/1 -> Demux1/1
  Pos dist/1 -> Demux2/1
  Demux2/1 -> Subsystem1/8(dx)
  Demux2/2 -> Subsystem/8(dy)
  Demux2/3 -> Subsystem2/7(dz)

== system CFBTTCQIED/Subsystem2/DO_params1 ==
  Pos rates : Inport
  Pos con Ux Uy Uz : Inport  Port=2
  Demux : Demux  Outputs=3
  Demux1 : Demux  Outputs=3
  Mux1 : Mux  Inputs=3
  Scope{,1..4} (5 alike) : Scope
  To Workspace : ToWorkspace  VariableName=pos_x_DO  SampleTime=-1
  To Workspace1 : ToWorkspace  VariableName=pos_y_DO  SampleTime=-1
  To Workspace2 : ToWorkspace  VariableName=pos_z_DO  SampleTime=-1
  pos x : Subsystem
  pos x1 : Subsystem
  pos x2 : Subsystem
  Pos DOs : Outport
  wires:
  Mux1/1 -> Pos DOs/1
  pos x/1(pos x do) -> To Workspace/1, Mux1/1, Scope/1
  pos x2/1(pos z do) -> Mux1/3, Scope2/1, To Workspace2/1
  Demux/1 -> Scope3/1, pos x/1(x8)
  Pos rates/1 -> Demux/1
  Pos con Ux Uy Uz/1 -> Demux1/1
  pos x1/1(pos y do) -> Mux1/2, Scope1/1, To Workspace1/1
  Demux1/1 -> Scope4/1, pos x/2(Ux)
  Demux/2 -> pos x1/1(x10)
  Demux1/2 -> pos x1/2(Uy)
  Demux/3 -> pos x2/1(x12)
  Demux1/3 -> pos x2/2(Uz)

== system CFBTTCQIED/Subsystem2/Subsystem ==
  pos_mu : Inport
  Demux : Demux  Outputs=3
  Gain{,1..5} (6 alike) : Gain  Gain=1/tau
  Integrator : Integrator  ZeroCross=off
  Integrator1 : Integrator
  Integrator2 : Integrator
  Mux : Mux  Inputs=3
  Sum{,1..5} (6 alike) : Sum  Inputs=|+-
  To Workspace : ToWorkspace  VariableName=filter_pos1  SampleTime=-1
  To Workspace1 : ToWorkspace  VariableName=filter_pos2  SampleTime=-1
  To Workspace2 : ToWorkspace  VariableName=filter_pos3  SampleTime=-1
  pos_xi : Outport
  wires:
  Integrator/1 -> Sum3/2, To Workspace/1, Sum/2
  Sum/1 -> Gain/1
  Gain/1 -> Integrator/1
  Sum1/1 -> Gain1/1
  Gain1/1 -> Integrator1/1
  Demux/2 -> Sum4/1, Sum1/1
  Integrator1/1 -> Sum1/2, To Workspace1/1, Sum4/2
  Sum2/1 -> Gain2/1
  Gain2/1 -> Integrator2/1
  Demux/3 -> Sum2/1, Sum5/1
  Integrator2/1 -> Sum2/2, To Workspace2/1, Sum5/2
  Demux/1 -> Sum3/1, Sum/1
  pos_mu/1 -> Demux/1
  Mux/1 -> pos_xi/1
  Sum3/1 -> Gain3/1
  Gain3/1 -> Mux/1
  Sum4/1 -> Gain4/1
  Gain4/1 -> Mux/2
  Gain5/1 -> Mux/3
  Sum5/1 -> Gain5/1

== system CFBTTCQIED/Quadrotor_Attitude_Model/Subsystem/Pitch_model ==
  T1 : Inport
  T3 : Inport  Port=2
  phi_dot  hat : Inport  Port=3
  "psi_dot hat " : Inport  Port=4
  pitch dist : Inport  Port=5
  Gain : Gain  Gain=b2
  Gain1 : Gain  Gain=a4*Omega_r
  Gain2 : Gain  Gain=a3
  Gain3 : Gain  Gain=b
  Gain4 : Gain  Gain=b
  Gain5 : Gain  Gain=a1_p/epsi
  Gain6 : Gain  Gain=a2_y/epsi^2
  Product : Product
  Sum : Sum  Inputs=+-++
  Sum1 : Sum  Inputs=+-
  Sum2 : Sum  Inputs=|++
  Sum3 : Sum  Inputs=|+-
  theta : Integrator  InitialCondition=init_cond_pitch
  theta_dot : Integrator
  theta_hat out : Outport
  theta_dot_hat out : Outport  Port=2
  wires:
  theta/1 -> Sum3/2, theta_hat out/1
  Gain1/1 -> Sum/2
  T3/1 -> Gain3/1
  Gain2/1 -> Sum/1
  phi_dot  hat/1 -> Product/2, Gain1/1
  theta_dot/1 -> Sum2/1, theta_dot_hat out/1
  Sum1/1 -> Gain/1
  Product/1 -> Gain2/1
  "psi_dot hat "/1 -> Product/1
  T1/1 -> Gain4/1
  Gain/1 -> Sum/3
  Sum/1 -> theta_dot/1
  Gain4/1 -> Sum1/1
  Gain3/1 -> Sum1/2
  Sum2/1 -> theta/1
  pitch dist/1 -> Sum3/1
  Sum3/1 -> Gain6/1, Gain5/1
  Gain5/1 -> Sum2/2
  Gain6/1 -> Sum/4

== system CFBTTCQIED/Quadrotor_Attitude_Model/Subsystem/Roll_Model ==
  T2 : Inport
  T4 : Inport  Port=2
  "Theta_dot hat " : Inport  Port=3
  "Psi_hat dot " : Inport  Port=4
  y = roll : Inport  Port=5
  Gain : Gain  Gain=b1
  Gain1 : Gain  Gain=a2*Omega_r
  Gain2 : Gain  Gain=a1
  Gain3 : Gain  Gain=b
  Gain4 : Gain  Gain=b
  Gain5 : Gain  Gain=a1_r/epsi
  Gain6 : Gain  Gain=a2_r/epsi^2
  Product : Product
  Sum : Sum  Inputs=++++
  Sum1 : Sum  Inputs=+-
  Sum2 : Sum  Inputs=|++
  Sum3 : Sum  Inputs=|+-
  phi : Integrator  InitialCondition=init_cond_roll
  phi_dot : Integrator
  Phi hat_out : Outport
  Phi_dot_hat out : Outport  Port=2
  wires:
  phi/1 -> Phi hat_out/1, Sum3/2
  Product/1 -> Gain2/1
  T2/1 -> Gain4/1
  Sum1/1 -> Gain/1
  "Theta_dot hat "/1 -> Product/2, Gain1/1
  Gain/1 -> Sum/3
  T4/1 -> Gain3/1
  phi_dot/1 -> Sum2/1, Phi_dot_hat out/1
  Gain2/1 -> Sum/1
  "Psi_hat dot "/1 -> Product/1
  Gain1/1 -> Sum/2
  Sum/1 -> phi_dot/1
  Gain3/1 -> Sum1/1
  Gain4/1 -> Sum1/2
  Sum2/1 -> phi/1
  y = roll/1 -> Sum3/1
  Gain5/1 -> Sum2/2
  Sum3/1 -> Gain6/1, Gain5/1
  Gain6/1 -> Sum/4

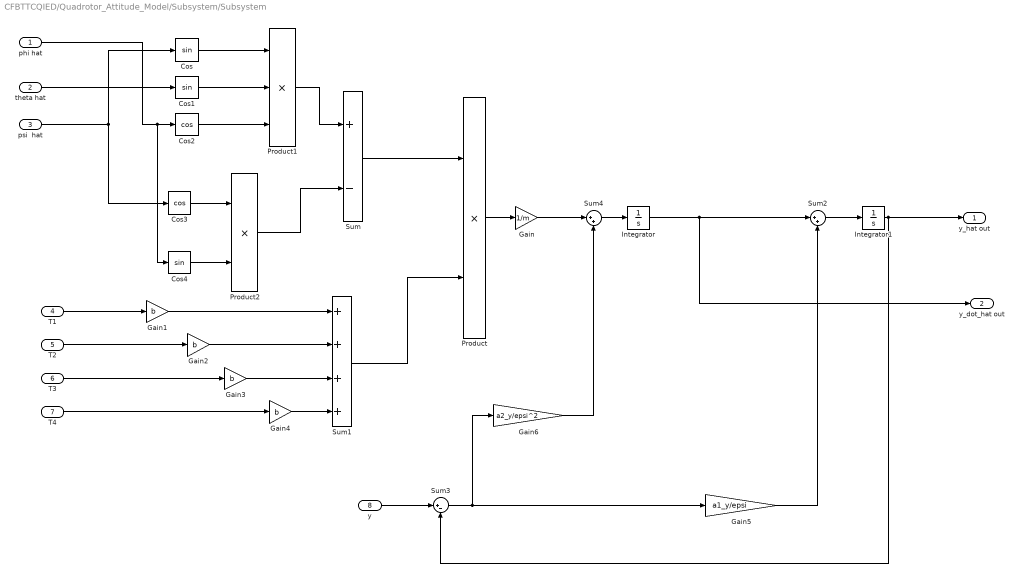
== system CFBTTCQIED/Quadrotor_Attitude_Model/Subsystem/Subsystem ==
  phi hat : Inport
  theta hat : Inport  Port=2
  psi  hat : Inport  Port=3
  T1 : Inport  Port=4
  T2 : Inport  Port=5
  T3 : Inport  Port=6
  T4 : Inport  Port=7
  y : Inport  Port=8
  Cos : Trigonometry
  Cos1 : Trigonometry
  Cos2 : Trigonometry  Operator=cos
  Cos3 : Trigonometry  Operator=cos
  Cos4 : Trigonometry
  Gain : Gain  Gain=1/m
  Gain{1..4} (4 alike) : Gain  Gain=b
  Gain5 : Gain  Gain=a1_y/epsi
  Gain6 : Gain  Gain=a2_y/epsi^2
  Integrator : Integrator
  Integrator1 : Integrator  InitialCondition=init_cond_y
  Product : Product
  Product1 : Product  Inputs=3
  Product2 : Product
  Sum : Sum  Inputs=+-
  Sum1 : Sum  Inputs=++++
  Sum2 : Sum  Inputs=|++
  Sum3 : Sum  Inputs=|+-
  Sum4 : Sum  Inputs=|++
  y_hat out : Outport
  y_dot_hat out : Outport  Port=2
  wires:
  Integrator/1 -> Sum2/1, y_dot_hat out/1
  Integrator1/1 -> Sum3/2, y_hat out/1
  Product/1 -> Gain/1
  Sum/1 -> Product/1
  Sum1/1 -> Product/2
  T2/1 -> Gain2/1
  T3/1 -> Gain3/1
  T4/1 -> Gain4/1
  T1/1 -> Gain1/1
  Gain1/1 -> Sum1/1
  Gain2/1 -> Sum1/2
  Gain3/1 -> Sum1/3
  Gain4/1 -> Sum1/4
  Product1/1 -> Sum/1
  Cos/1 -> Product1/1
  Cos2/1 -> Product1/3
  Product2/1 -> Sum/2
  Cos1/1 -> Product1/2
  Cos3/1 -> Product2/1
  Cos4/1 -> Product2/2
  psi  hat/1 -> Cos3/1, Cos/1
  theta hat/1 -> Cos1/1
  phi hat/1 -> Cos4/1, Cos2/1
  Sum2/1 -> Integrator1/1
  y/1 -> Sum3/1
  Sum3/1 -> Gain6/1, Gain5/1
  Gain5/1 -> Sum2/2
  Sum4/1 -> Integrator/1
  Gain/1 -> Sum4/1
  Gain6/1 -> Sum4/2

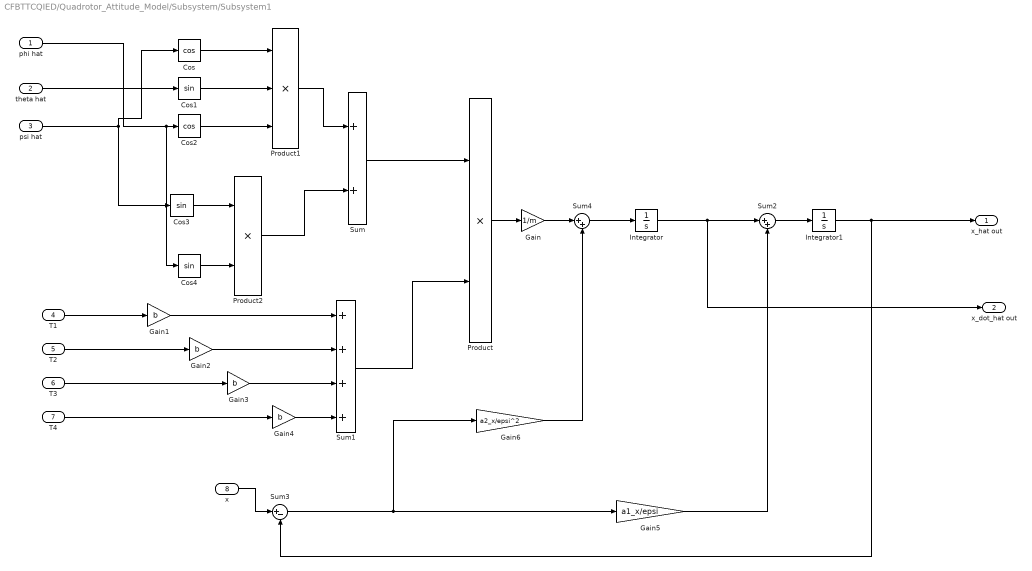
== system CFBTTCQIED/Quadrotor_Attitude_Model/Subsystem/Subsystem1 ==
  phi hat : Inport
  theta hat : Inport  Port=2
  psi hat : Inport  Port=3
  T1 : Inport  Port=4
  T2 : Inport  Port=5
  T3 : Inport  Port=6
  T4 : Inport  Port=7
  x : Inport  Port=8
  Cos : Trigonometry  Operator=cos
  Cos1 : Trigonometry
  Cos2 : Trigonometry  Operator=cos
  Cos3 : Trigonometry
  Cos4 : Trigonometry
  Gain : Gain  Gain=1/m
  Gain{1..4} (4 alike) : Gain  Gain=b
  Gain5 : Gain  Gain=a1_x/epsi
  Gain6 : Gain  Gain=a2_x/epsi^2
  Integrator : Integrator
  Integrator1 : Integrator  InitialCondition=init_cond_x
  Product : Product
  Product1 : Product  Inputs=3
  Product2 : Product
  Sum : Sum
  Sum1 : Sum  Inputs=++++
  Sum2 : Sum  Inputs=|++
  Sum3 : Sum  Inputs=|+-
  Sum4 : Sum  Inputs=|++
  x_hat out : Outport
  x_dot_hat out : Outport  Port=2
  wires:
  Integrator/1 -> Sum2/1, x_dot_hat out/1
  Integrator1/1 -> Sum3/2, x_hat out/1
  Product/1 -> Gain/1
  Sum/1 -> Product/1
  Sum1/1 -> Product/2
  T2/1 -> Gain2/1
  T3/1 -> Gain3/1
  T4/1 -> Gain4/1
  T1/1 -> Gain1/1
  Gain1/1 -> Sum1/1
  Gain2/1 -> Sum1/2
  Gain3/1 -> Sum1/3
  Gain4/1 -> Sum1/4
  Product1/1 -> Sum/1
  Cos/1 -> Product1/1
  Cos2/1 -> Product1/3
  Product2/1 -> Sum/2
  Cos1/1 -> Product1/2
  Cos3/1 -> Product2/1
  Cos4/1 -> Product2/2
  psi hat/1 -> Cos/1, Cos3/1
  theta hat/1 -> Cos1/1
  phi hat/1 -> Cos4/1, Cos2/1
  Sum2/1 -> Integrator1/1
  x/1 -> Sum3/1
  Sum4/1 -> Integrator/1
  Gain/1 -> Sum4/1
  Sum3/1 -> Gain6/1, Gain5/1
  Gain5/1 -> Sum2/2
  Gain6/1 -> Sum4/2

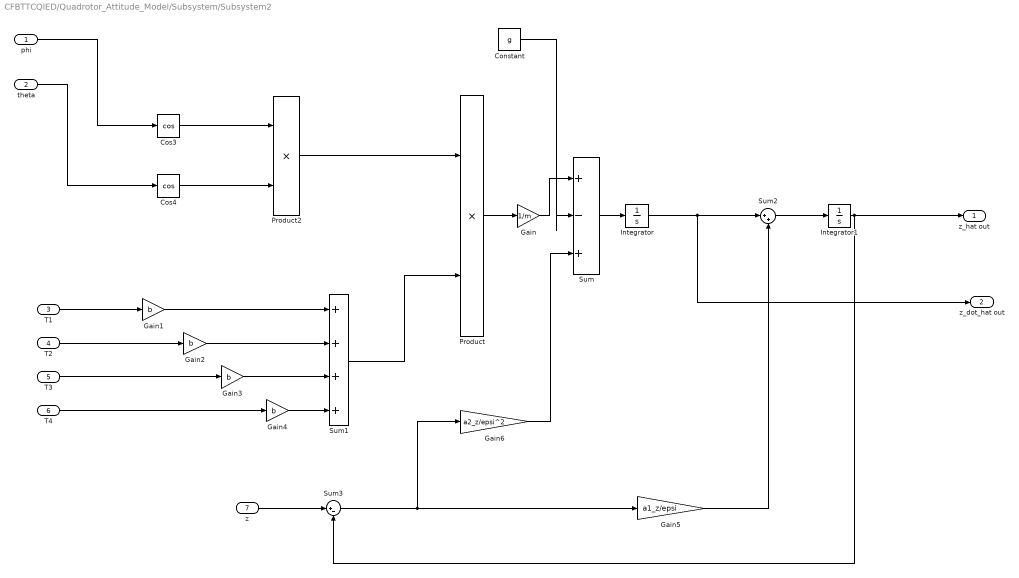
== system CFBTTCQIED/Quadrotor_Attitude_Model/Subsystem/Subsystem2 ==
  phi : Inport
  theta : Inport  Port=2
  T1 : Inport  Port=3
  T2 : Inport  Port=4
  T3 : Inport  Port=5
  T4 : Inport  Port=6
  z : Inport  Port=7
  Constant : Constant  Value=g
  Cos3 : Trigonometry  Operator=cos
  Cos4 : Trigonometry  Operator=cos
  Gain : Gain  Gain=1/m
  Gain{1..4} (4 alike) : Gain  Gain=b
  Gain5 : Gain  Gain=a1_z/epsi
  Gain6 : Gain  Gain=a2_z/epsi^2
  Integrator : Integrator
  Integrator1 : Integrator  InitialCondition=init_cond_z
  Product : Product
  Product2 : Product
  Sum : Sum  Inputs=|+-+
  Sum1 : Sum  Inputs=++++
  Sum2 : Sum  Inputs=|++
  Sum3 : Sum  Inputs=|+-
  z_hat out : Outport
  z_dot_hat out : Outport  Port=2
  wires:
  Integrator/1 -> Sum2/1, z_dot_hat out/1
  Integrator1/1 -> Sum3/2, z_hat out/1
  Product/1 -> Gain/1
  Sum1/1 -> Product/2
  T2/1 -> Gain2/1
  T3/1 -> Gain3/1
  T4/1 -> Gain4/1
  T1/1 -> Gain1/1
  Gain1/1 -> Sum1/1
  Gain2/1 -> Sum1/2
  Gain3/1 -> Sum1/3
  Gain4/1 -> Sum1/4
  Cos3/1 -> Product2/1
  Cos4/1 -> Product2/2
  Product2/1 -> Product/1
  phi/1 -> Cos3/1
  theta/1 -> Cos4/1
  Gain/1 -> Sum/1
  Sum/1 -> Integrator/1
  Constant/1 -> Sum/2
  Sum2/1 -> Integrator1/1
  z/1 -> Sum3/1
  Gain5/1 -> Sum2/2
  Gain6/1 -> Sum/3
  Sum3/1 -> Gain6/1, Gain5/1

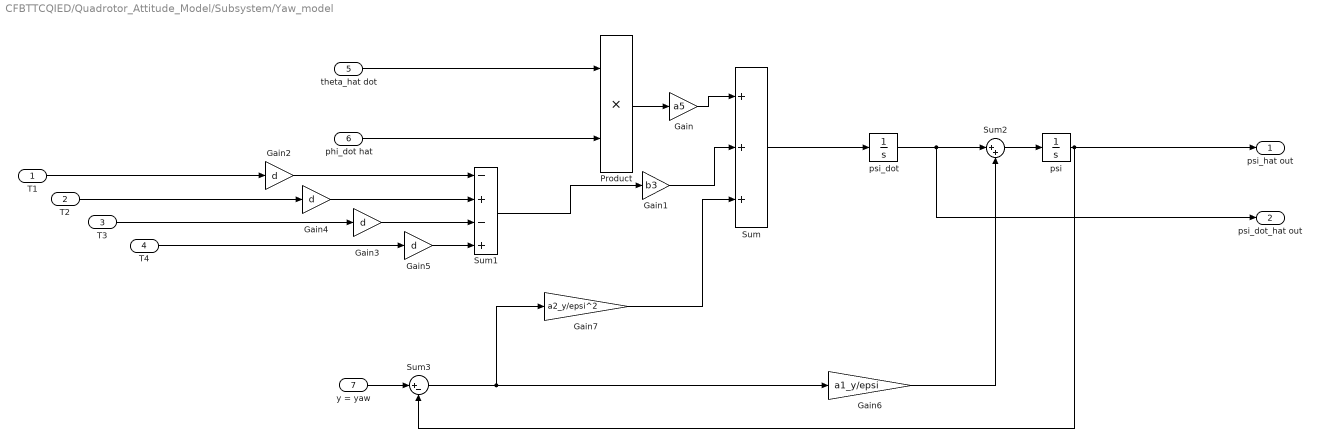
== system CFBTTCQIED/Quadrotor_Attitude_Model/Subsystem/Yaw_model ==
  " T1" : Inport
  T2 : Inport  Port=2
  T3 : Inport  Port=3
  T4 : Inport  Port=4
  "theta_hat dot " : Inport  Port=5
  "phi_dot hat  " : Inport  Port=6
  y = yaw : Inport  Port=7
  Gain : Gain  Gain=a5
  Gain1 : Gain  Gain=b3
  Gain{2..5} (4 alike) : Gain  Gain=d
  Gain6 : Gain  Gain=a1_y/epsi
  Gain7 : Gain  Gain=a2_y/epsi^2
  Product : Product
  Sum : Sum  Inputs=+++
  Sum1 : Sum  Inputs=-+-+
  Sum2 : Sum  Inputs=|++
  Sum3 : Sum  Inputs=|+-
  psi : Integrator  InitialCondition=init_cond_yaw
  psi_dot : Integrator
  psi_hat out : Outport
  psi_dot_hat out : Outport  Port=2
  wires:
  Product/1 -> Gain/1
  psi/1 -> Sum3/2, psi_hat out/1
  "theta_hat dot "/1 -> Product/1
  psi_dot/1 -> Sum2/1, psi_dot_hat out/1
  T3/1 -> Gain3/1
  Sum1/1 -> Gain1/1
  Sum/1 -> psi_dot/1
  Gain1/1 -> Sum/2
  Gain/1 -> Sum/1
  "phi_dot hat  "/1 -> Product/2
  " T1"/1 -> Gain2/1
  T2/1 -> Gain4/1
  T4/1 -> Gain5/1
  Gain2/1 -> Sum1/1
  Gain4/1 -> Sum1/2
  Gain3/1 -> Sum1/3
  Gain5/1 -> Sum1/4
  Sum2/1 -> psi/1
  y = yaw/1 -> Sum3/1
  Sum3/1 -> Gain7/1, Gain6/1
  Gain6/1 -> Sum2/2
  Gain7/1 -> Sum/3

== system CFBTTCQIED/Quadrotor_Attitude_Model/Subsystem3/Pitch_model ==
  note: inpt
  T1 : Inport
  T3 : Inport  Port=2
  "phi_dot " : Inport  Port=3
  "psi_dot " : Inport  Port=4
  pitch dist : Inport  Port=5
  Gain : Gain  Gain=b2
  Gain1 : Gain  Gain=a4*Omega_r
  Gain2 : Gain  Gain=a3
  Gain3 : Gain  Gain=b
  Gain4 : Gain  Gain=b
  Product : Product
  Sum : Sum  Inputs=+-++
  Sum1 : Sum  Inputs=+-
  theta : Integrator  InitialCondition=init_cond_pitch
  theta_dot : Integrator
  theta_out : Outport
  theta_dot_out : Outport  Port=2
  wires:
  theta/1 -> theta_out/1
  Gain1/1 -> Sum/2
  T3/1 -> Gain3/1
  Gain2/1 -> Sum/1
  "phi_dot "/1 -> Product/2, Gain1/1
  theta_dot/1 -> theta_dot_out/1, theta/1
  Sum1/1 -> Gain/1
  Product/1 -> Gain2/1
  "psi_dot "/1 -> Product/1
  T1/1 -> Gain4/1
  Gain/1 -> Sum/3
  Sum/1 -> theta_dot/1
  Gain4/1 -> Sum1/1
  Gain3/1 -> Sum1/2
  pitch dist/1 -> Sum/4

== system CFBTTCQIED/Quadrotor_Attitude_Model/Subsystem3/Roll_Model ==
  T2 : Inport
  T4 : Inport  Port=2
  "Theta_dot " : Inport  Port=3
  "Psi_dot " : Inport  Port=4
  roll dist : Inport  Port=5
  Gain : Gain  Gain=b1
  Gain1 : Gain  Gain=a2*Omega_r
  Gain2 : Gain  Gain=a1
  Gain3 : Gain  Gain=b
  Gain4 : Gain  Gain=b
  Product : Product
  Sum : Sum  Inputs=++++
  Sum1 : Sum  Inputs=+-
  phi : Integrator  InitialCondition=init_cond_roll
  phi_dot : Integrator
  Phi_out : Outport
  Phi_dot_out : Outport  Port=2
  wires:
  phi/1 -> Phi_out/1
  Product/1 -> Gain2/1
  T2/1 -> Gain4/1
  Sum1/1 -> Gain/1
  "Theta_dot "/1 -> Product/2, Gain1/1
  Gain/1 -> Sum/3
  T4/1 -> Gain3/1
  phi_dot/1 -> Phi_dot_out/1, phi/1
  Gain2/1 -> Sum/1
  "Psi_dot "/1 -> Product/1
  Gain1/1 -> Sum/2
  Sum/1 -> phi_dot/1
  Gain3/1 -> Sum1/1
  Gain4/1 -> Sum1/2
  roll dist/1 -> Sum/4

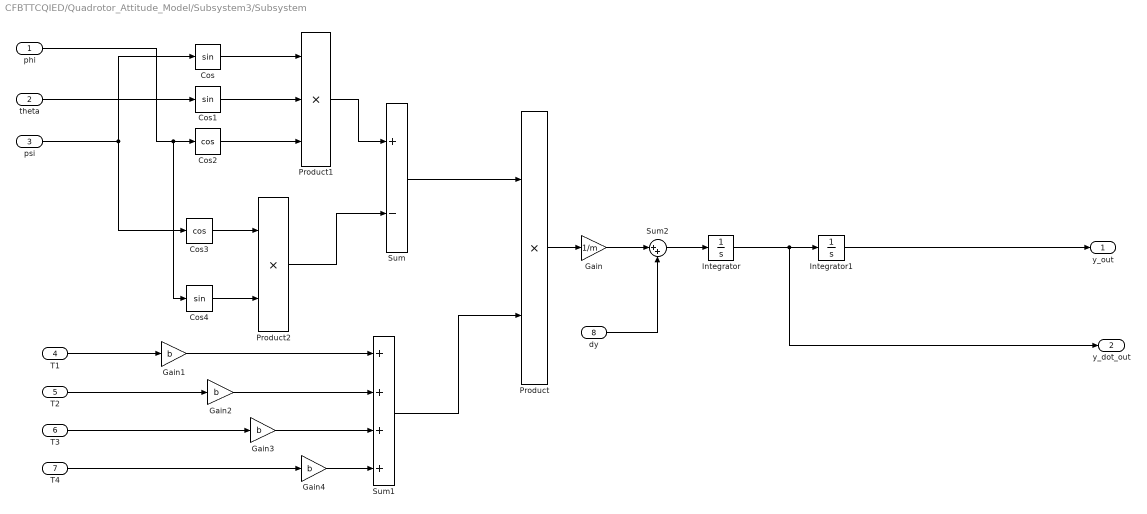
== system CFBTTCQIED/Quadrotor_Attitude_Model/Subsystem3/Subsystem ==
  phi : Inport
  theta : Inport  Port=2
  psi : Inport  Port=3
  T1 : Inport  Port=4
  T2 : Inport  Port=5
  T3 : Inport  Port=6
  T4 : Inport  Port=7
  dy : Inport  Port=8
  Cos : Trigonometry
  Cos1 : Trigonometry
  Cos2 : Trigonometry  Operator=cos
  Cos3 : Trigonometry  Operator=cos
  Cos4 : Trigonometry
  Gain : Gain  Gain=1/m
  Gain{1..4} (4 alike) : Gain  Gain=b
  Integrator : Integrator
  Integrator1 : Integrator  InitialCondition=init_cond_y
  Product : Product
  Product1 : Product  Inputs=3
  Product2 : Product
  Sum : Sum  Inputs=+-
  Sum1 : Sum  Inputs=++++
  Sum2 : Sum  Inputs=|++
  y_out : Outport
  y_dot_out : Outport  Port=2
  wires:
  Integrator/1 -> y_dot_out/1, Integrator1/1
  Integrator1/1 -> y_out/1
  Product/1 -> Gain/1
  Sum/1 -> Product/1
  Sum1/1 -> Product/2
  T2/1 -> Gain2/1
  T3/1 -> Gain3/1
  T4/1 -> Gain4/1
  T1/1 -> Gain1/1
  Gain1/1 -> Sum1/1
  Gain2/1 -> Sum1/2
  Gain3/1 -> Sum1/3
  Gain4/1 -> Sum1/4
  Product1/1 -> Sum/1
  Cos/1 -> Product1/1
  Cos2/1 -> Product1/3
  Product2/1 -> Sum/2
  Cos1/1 -> Product1/2
  Cos3/1 -> Product2/1
  Cos4/1 -> Product2/2
  psi/1 -> Cos3/1, Cos/1
  theta/1 -> Cos1/1
  phi/1 -> Cos4/1, Cos2/1
  Sum2/1 -> Integrator/1
  Gain/1 -> Sum2/1
  dy/1 -> Sum2/2

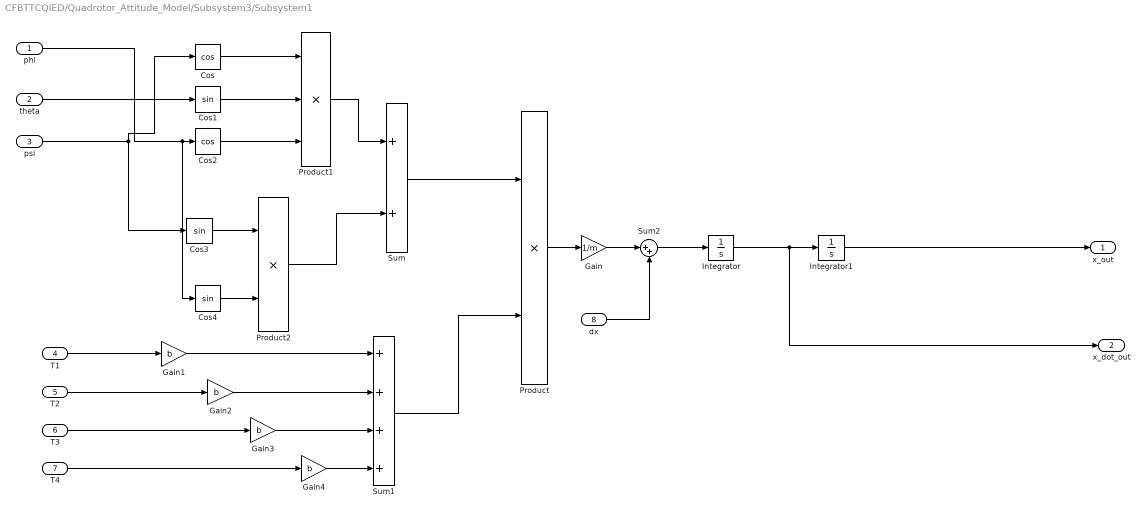
== system CFBTTCQIED/Quadrotor_Attitude_Model/Subsystem3/Subsystem1 ==
  phi : Inport
  theta : Inport  Port=2
  psi : Inport  Port=3
  T1 : Inport  Port=4
  T2 : Inport  Port=5
  T3 : Inport  Port=6
  T4 : Inport  Port=7
  dx : Inport  Port=8
  Cos : Trigonometry  Operator=cos
  Cos1 : Trigonometry
  Cos2 : Trigonometry  Operator=cos
  Cos3 : Trigonometry
  Cos4 : Trigonometry
  Gain : Gain  Gain=1/m
  Gain{1..4} (4 alike) : Gain  Gain=b
  Integrator : Integrator
  Integrator1 : Integrator  InitialCondition=init_cond_x
  Product : Product
  Product1 : Product  Inputs=3
  Product2 : Product
  Sum : Sum
  Sum1 : Sum  Inputs=++++
  Sum2 : Sum  Inputs=|++
  x_out : Outport
  x_dot_out : Outport  Port=2
  wires:
  Integrator/1 -> x_dot_out/1, Integrator1/1
  Integrator1/1 -> x_out/1
  Product/1 -> Gain/1
  Sum/1 -> Product/1
  Sum1/1 -> Product/2
  T2/1 -> Gain2/1
  T3/1 -> Gain3/1
  T4/1 -> Gain4/1
  T1/1 -> Gain1/1
  Gain1/1 -> Sum1/1
  Gain2/1 -> Sum1/2
  Gain3/1 -> Sum1/3
  Gain4/1 -> Sum1/4
  Product1/1 -> Sum/1
  Cos/1 -> Product1/1
  Cos2/1 -> Product1/3
  Product2/1 -> Sum/2
  Cos1/1 -> Product1/2
  Cos3/1 -> Product2/1
  Cos4/1 -> Product2/2
  psi/1 -> Cos/1, Cos3/1
  theta/1 -> Cos1/1
  phi/1 -> Cos4/1, Cos2/1
  Gain/1 -> Sum2/1
  Sum2/1 -> Integrator/1
  dx/1 -> Sum2/2

== system CFBTTCQIED/Quadrotor_Attitude_Model/Subsystem3/Subsystem2 ==
  phi : Inport
  theta : Inport  Port=2
  T1 : Inport  Port=3
  T2 : Inport  Port=4
  T3 : Inport  Port=5
  T4 : Inport  Port=6
  dz : Inport  Port=7
  Constant : Constant  Value=g
  Cos3 : Trigonometry  Operator=cos
  Cos4 : Trigonometry  Operator=cos
  Gain : Gain  Gain=1/m
  Gain{1..4} (4 alike) : Gain  Gain=b
  Integrator : Integrator
  Integrator1 : Integrator  InitialCondition=init_cond_z
  Product : Product
  Product2 : Product
  Sum : Sum  Inputs=-++
  Sum1 : Sum  Inputs=++++
  z_out : Outport
  z_dot_out : Outport  Port=2
  wires:
  Integrator/1 -> z_dot_out/1, Integrator1/1
  Integrator1/1 -> z_out/1
  Product/1 -> Gain/1
  Sum1/1 -> Product/2
  T2/1 -> Gain2/1
  T3/1 -> Gain3/1
  T4/1 -> Gain4/1
  T1/1 -> Gain1/1
  Gain1/1 -> Sum1/1
  Gain2/1 -> Sum1/2
  Gain3/1 -> Sum1/3
  Gain4/1 -> Sum1/4
  Cos3/1 -> Product2/1
  Cos4/1 -> Product2/2
  Product2/1 -> Product/1
  phi/1 -> Cos3/1
  theta/1 -> Cos4/1
  Sum/1 -> Integrator/1
  Gain/1 -> Sum/2
  Constant/1 -> Sum/1
  dz/1 -> Sum/3

== system CFBTTCQIED/Quadrotor_Attitude_Model/Subsystem3/Yaw_model ==
  " T1" : Inport
  T2 : Inport  Port=2
  T3 : Inport  Port=3
  T4 : Inport  Port=4
  "theta_dot " : Inport  Port=5
  "phi_dot " : Inport  Port=6
  yaw dist : Inport  Port=7
  Gain : Gain  Gain=a5
  Gain1 : Gain  Gain=b3
  Gain{2..5} (4 alike) : Gain  Gain=d
  Product : Product
  Sum : Sum  Inputs=+++
  Sum1 : Sum  Inputs=-+-+
  psi : Integrator  InitialCondition=init_cond_yaw
  psi_dot : Integrator
  psi_out : Outport
  psi_dot_out : Outport  Port=2
  wires:
  Product/1 -> Gain/1
  psi/1 -> psi_out/1
  "theta_dot "/1 -> Product/1
  psi_dot/1 -> psi_dot_out/1, psi/1
  T3/1 -> Gain3/1
  Sum1/1 -> Gain1/1
  Sum/1 -> psi_dot/1
  Gain1/1 -> Sum/2
  Gain/1 -> Sum/1
  "phi_dot "/1 -> Product/2
  " T1"/1 -> Gain2/1
  T2/1 -> Gain4/1
  T4/1 -> Gain5/1
  Gain2/1 -> Sum1/1
  Gain4/1 -> Sum1/2
  Gain3/1 -> Sum1/3
  Gain5/1 -> Sum1/4
  yaw dist/1 -> Sum/3

== system CFBTTCQIED/Subsystem2/DO_params1/pos x ==
  x8 : Inport
  Ux : Inport  Port=2
  Gain1 : Gain  Gain=lambda_x
  Gain4 : Gain  Gain=lambda_x
  Gain5 : Gain  Gain=lambda_x*lambda_x
  Gain9 : Gain  Gain=lambda_x
  Integrator2 : Integrator
  Scope{,1..4} (5 alike) : Scope
  Sum1 : Sum
  Sum4 : Sum  Inputs=---
  pos x do : Outport
  wires:
  x8/1 -> Scope1/1, Gain9/1, Gain5/1
  Gain4/1 -> Sum4/1
  Gain5/1 -> Sum4/2
  Sum4/1 -> Integrator2/1
  Integrator2/1 -> Sum1/1, Scope/1, Gain4/1
  Gain9/1 -> Scope3/1, Sum1/2
  Sum1/1 -> pos x do/1
  Gain1/1 -> Scope4/1, Sum4/3
  Ux/1 -> Scope2/1, Gain1/1

== system CFBTTCQIED/Subsystem2/DO_params1/pos x1 ==
  x10 : Inport
  Uy : Inport  Port=2
  Gain1 : Gain  Gain=lambda_y
  Gain4 : Gain  Gain=lambda_y
  Gain5 : Gain  Gain=lambda_y*lambda_y
  Gain9 : Gain  Gain=lambda_y
  Integrator2 : Integrator
  Scope : Scope
  Sum1 : Sum
  Sum4 : Sum  Inputs=---
  pos y do : Outport
  wires:
  Uy/1 -> Gain1/1
  Gain1/1 -> Sum4/3
  Sum1/1 -> pos y do/1
  Gain9/1 -> Sum1/2
  Integrator2/1 -> Gain4/1, Scope/1, Sum1/1
  Sum4/1 -> Integrator2/1
  Gain5/1 -> Sum4/2
  Gain4/1 -> Sum4/1
  x10/1 -> Gain5/1, Gain9/1

== system CFBTTCQIED/Subsystem2/DO_params1/pos x2 ==
  x12 : Inport
  Uz : Inport  Port=2
  Gain1 : Gain  Gain=lambda_z
  Gain4 : Gain  Gain=lambda_z
  Gain5 : Gain  Gain=lambda_z*lambda_z
  Gain9 : Gain  Gain=lambda_z
  Integrator2 : Integrator
  Scope : Scope
  Sum1 : Sum
  Sum4 : Sum  Inputs=---
  pos z do : Outport
  wires:
  x12/1 -> Gain9/1, Gain5/1
  Gain4/1 -> Sum4/1
  Gain5/1 -> Sum4/2
  Sum4/1 -> Integrator2/1
  Integrator2/1 -> Sum1/1, Scope/1, Gain4/1
  Gain9/1 -> Sum1/2
  Sum1/1 -> pos z do/1
  Gain1/1 -> Sum4/3
  Uz/1 -> Gain1/1

== matlab function CFBTTCQIED/Trajectory/MATLAB Function2 ==
  data: t input; x_des output; y_des output; z_des output
function [x_des,y_des,z_des] = fcn(t)
x_des = 3 - 3*cos(t/15);
y_des = 2 + 3*sin(t/15);
z_des = 2 + 0.10*t;
%x_des =0;
%y_des =0;
%z_des = 5;
y = [x_des,y_des,z_des] ;

== matlab function CFBTTCQIED/Quadrotor_Attitude_Model/Motor Dynamics ==
  data: U1 input; T1 output; T2 output; T3 output; T4 output; U2 input; U3 input; U4 input
function [T1,T2,T3,T4] = fcn(U1,U2,U3,U4)

%params 
b = 3.13e-5;             % Thrust coefficient         [N.sec^2]
d = 7.5e-7;              % Drag coefficient           [Nm.sec^2]

%Control mixing

T1 = U1/(4*b)       +0              +U3/(2*b)           -U4/(4*d);
T2 = U1/(4*b)       -U2/(2*b)       +0                  +U4/(4*d);
T3 = U1/(4*b)       +0              -U3/(2*b)           -U4/(4*d);
T4 = U1/(4*b)       +U2/(2*b)       +0                  +U4/(4*d);

y = [T1,T2,T3,T4];

== matlab function CFBTTCQIED/Subsystem2/MATLAB Function ==
  data: Ux input; U1 output; Uy input; Uz input; psi_des input; theta_des output; phi_des output
function [U1,theta_des,phi_des] = fcn(Ux,Uy,Uz,psi_des)
% Parameters
g = 9.81;                % Gravity                    [m/sec^2]     
m = 0.650;               % Mass                       [kg]     
l = 0.23;                % Length                     [m]
k = 2.980e-6;            %
b = 3.13e-5;             % Thrust coefficient         [N.sec^2]
d = 7.5e-7;              % Drag coefficient           [Nm.sec^2]
R_rad = 0.15;            % Properller radius          [m]
c = 0.04;                % Properller chord           [m]
Jr = 6e-5;               % Rotor inertia              [kg.m^2]

Im = 3.357e-5;           %
Ixx = 7.5e-3;            % Inertia on x-axis          [kg.m^2]
Iyy = 7.5e-3;            % Inertia on y-axis          [kg.m^2]
Izz = 1.3e-2;            % Inertia on z-axis          [kg.m^2]

Omega_r = 1;             % Residual angular speed of propeller     [rad.sec]
% Parameters simplification
a1 = (Iyy-Izz)/Ixx;
a2 = Jr/Ixx;
b1 = l/Ixx;


a3 = (Izz-Ixx)/Iyy;
a4 = Jr/Iyy;
b2 = l/Iyy;

a5 = (Ixx-Iyy)/Izz;
b3 = l/Izz;
%%
% Desired roll, pitch and yaw
theta_des = atan((cos(psi_des)*Ux + sin(psi_des)*Uy)/(Uz+g));
phi_des = atan((sin(psi_des)*Ux - cos(psi_des)*Uy)*cos(theta_des)/(Uz+g));

% Controller
U1 = (m*(Uz+g))/(cos(phi_des)*cos(theta_des));

y = [U1,theta_des,phi_des];
